simulink model "motorPWM"  (R2021b)
settings: Solver=VariableStepAuto  StartTime=0.0  StopTime=10.0  RelTol=1e-3
values from neighbouring files (symbols this model uses):
  b = 0.5    [Assignment2_Curtis.m]    (also in Assignment2m_Curtis.m)
  J = 0.05    [Assignment2_Curtis.m]    (also in Assignment2m_Curtis.m)
  Ke = 0.5    [Assignment2_Curtis.m]    (also in Assignment2m_Curtis.m)
  Kt = 0.5    [Assignment2_Curtis.m]    (also in Assignment2m_Curtis.m)
  Ra = 1    [Assignment2_Curtis.m]    (also in Assignment2m_Curtis.m)
libraries: simulink x2
settings Model: Creator=Alex  LastModifiedBy=Alex

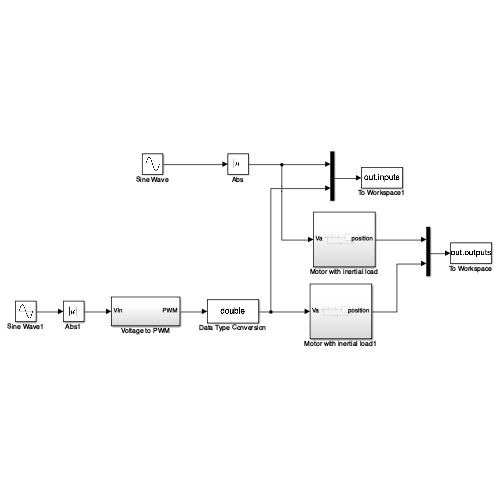
[thumbnail: Simulink's stored preview of the top-level diagram]
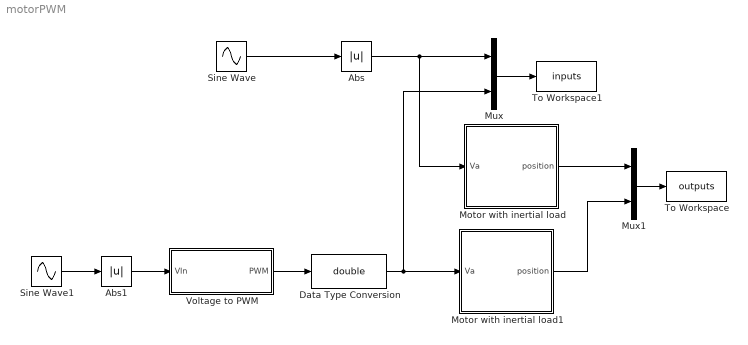
== system motorPWM ==
  Abs : Abs
  Abs1 : Abs
  Data Type Conversion : DataTypeConversion  OutDataTypeStr=double
  Motor with inertial load : Subsystem
  Motor with inertial load1 : Subsystem
  Mux : Mux  Inputs=2
  Mux1 : Mux  Inputs=2
  Sine Wave : Sin  SampleTime=0
  Sine Wave1 : Sin  SampleTime=0
  To Workspace : ToWorkspace  VariableName=outputs  SaveFormat=Timeseries  SampleTime=-1
  To Workspace1 : ToWorkspace  VariableName=inputs  SaveFormat=Timeseries  SampleTime=-1
  Voltage to PWM : Subsystem
  wires:
  Abs/1 -> Motor with inertial load/1(Va), Mux/1
  Sine Wave/1 -> Abs/1
  Motor with inertial load/1(position) -> Mux1/1
  Abs1/1 -> Voltage to PWM/1(VIn)
  Voltage to PWM/1(PWM) -> Data Type Conversion/1
  Sine Wave1/1 -> Abs1/1
  Motor with inertial load1/1(position) -> Mux1/2
  Data Type Conversion/1 -> Motor with inertial load1/1(Va), Mux/2
  Mux1/1 -> To Workspace/1
  Mux/1 -> To Workspace1/1

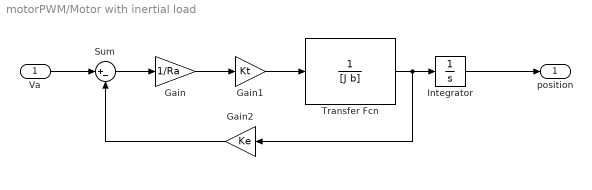
== system motorPWM/Motor with inertial load ==
  Va : Inport
  Gain : Gain  Gain=1/Ra
  Gain1 : Gain  Gain=Kt
  Gain2 : Gain  Gain=Ke
  Integrator : Integrator
  Sum : Sum  Inputs=|+-
  Transfer Fcn : TransferFcn  Denominator=[J b]
  position : Outport
  wires:
  Va/1 -> Sum/1
  Integrator/1 -> position/1
  Sum/1 -> Gain/1
  Gain/1 -> Gain1/1
  Gain2/1 -> Sum/2
  Transfer Fcn/1 -> Integrator/1, Gain2/1
  Gain1/1 -> Transfer Fcn/1

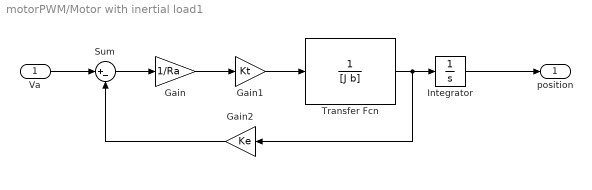
== system motorPWM/Motor with inertial load1 ==
  Va : Inport
  Gain : Gain  Gain=1/Ra
  Gain1 : Gain  Gain=Kt
  Gain2 : Gain  Gain=Ke
  Integrator : Integrator
  Sum : Sum  Inputs=|+-
  Transfer Fcn : TransferFcn  Denominator=[J b]
  position : Outport
  wires:
  Va/1 -> Sum/1
  Integrator/1 -> position/1
  Sum/1 -> Gain/1
  Gain/1 -> Gain1/1
  Gain2/1 -> Sum/2
  Transfer Fcn/1 -> Integrator/1, Gain2/1
  Gain1/1 -> Transfer Fcn/1

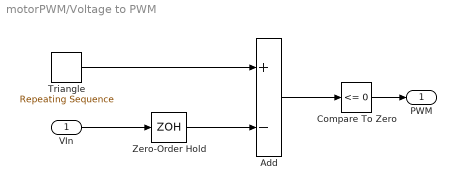
== system motorPWM/Voltage to PWM ==
  VIn : Inport
  Add : Sum  Inputs=+-  SampleTime=1/10000
  Compare To Zero : simulink/Logic and Bit Operations/Compare To Zero  relop=<=  OutDataTypeStr=uint8
  Triangle : simulink/Sources/Repeating Sequence  rep_seq_t=[0 1/100/4 3/100/4 1/100]*25  rep_seq_y=[0.5 0 1 0.5]
  Zero-Order Hold : ZeroOrderHold  SampleTime=1/10000
  PWM : Outport  VectorParamsAs1DForOutWhenUnconnected=off
  wires:
  Triangle/1 -> Add/1
  VIn/1 -> Zero-Order Hold/1
  Add/1 -> Compare To Zero/1
  Compare To Zero/1 -> PWM/1
  Zero-Order Hold/1 -> Add/2
